simulink model "arrayheattransfersimulinkmodel"  (R2023b)
settings: Solver=VariableStepAuto  StartTime=0.0  StopTime=10.0  RelTol=1e-3
settings Model: Creator=Tom Cruise  LastModifiedBy=Tom Cruise

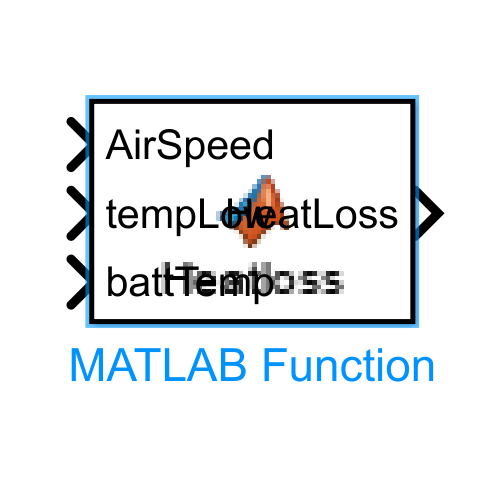
[thumbnail: Simulink's stored preview of the top-level diagram]
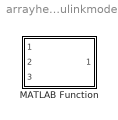
== system arrayheattransfersimulinkmodel ==
  MATLAB Function : MATLAB Function  TreatAsAtomicUnit=on

== matlab function arrayheattransfersimulinkmodel/MATLAB Function ==
  data: AirSpeed input; HeatLoss output; tempLow input; battTemp input




function HeatLoss = Heatloss(AirSpeed,tempLow,battTemp)
addpath('path_to_coolprop_folder');

%Reynolds Number Calcs
    BattColumns = 5;
    BatteryRows =23;
    
    tempHigh = 40 + 273.15;
    DiameterCells = 18.3/1000; % CHANGE THIS BECAUSE NO GAP




    dynViscosity = py.CoolProp.CoolProp.PropsSI('V', 'T', tempLow, 'P|not_imposed', 101325, 'air');
    densityAir = py.CoolProp.CoolProp.PropsSI('D', 'T', tempLow, 'P|not_imposed', 101325, 'air')
    thermCond = py.CoolProp.CoolProp.PropsSI('L', 'T', tempLow, 'P|not_imposed', 101325, 'air');
    ConstPNum = py.CoolProp.CoolProp.PropsSI('C', 'T', tempLow, 'P|not_imposed', 101325, 'air');
    thermMassAir = py.CoolProp.CoolProp.PropsSI('C', 'T', tempLow, 'P|not_imposed', 101325, 'air')
    KinViscosity = dynViscosity/densityAir;


% Vert vs Horiz Spacing
    St = 24.3/1000;% spacing between columns
    Sl = 34.3/1000;%center spacing in direction of initial airflow
    
    Vmax =  St.*AirSpeed./(St-DiameterCells);

    ReynoldsNumber =  Vmax * DiameterCells / KinViscosity % WILL have to update C1 and M Manually before IF statements. 
    PrandtlAirLow = py.CoolProp.CoolProp.PropsSI('Prandtl', 'T', tempLow, 'P|not_imposed', 101325, 'air');
    PrandtlAirHigh = py.CoolProp.CoolProp.PropsSI('Prandtl', 'T', tempHigh, 'P|not_imposed', 101325, 'air');

    C1 = 0.35*(St/Sl)^(1/5);
    mVal = 0.6; % Table
    C2 = 0.95; %Table (correction factor for 5)





    NusseltD = C2*C1*ReynoldsNumber.^mVal.*(PrandtlAirLow.^0.36).*(PrandtlAirLow./PrandtlAirHigh).^(0.25);
    Hline = NusseltD*thermCond/DiameterCells;







    insideVarTop = (-pi*DiameterCells*(BattColumns*BatteryRows)*Hline);

    insideVarBot = (densityAir.*AirSpeed.*(BatteryRows)*St*ConstPNum);
    adjDelTso = (battTemp - tempLow) * exp(insideVarTop/insideVarBot);
    To = -((battTemp - tempLow) * exp(insideVarTop/insideVarBot))+battTemp -273.15


    deltTlm = ((battTemp-tempLow)-(adjDelTso))/(log((battTemp-tempLow)/(adjDelTso)));

    qPrime = (BatteryRows*BattColumns)*(Hline*pi*DiameterCells*deltTlm);%in KW per m
    qPrimeLadjust = qPrime*0.065*6%Temp dissapated
    areaPath = St*BattColumns*0.065;


    Pt = St/DiameterCells;
    Pl = Sl/DiameterCells;
    PTPL = (Pt-1)/(Pl-1);

    fancyX = 1.4;
    fricFactor = 0.22;

    deltPLoss = 5.* fancyX .* (densityAir./2.*Vmax.^2) .* fricFactor;

    HeatLoss = qPrimeLadjust;

end
